simulink model "PHRI_MODEL_PROJECT"  (R2020b)
settings: Solver=VariableStepAuto  StartTime=0.0  StopTime=20  RelTol=1e-3
values from neighbouring files (symbols this model uses):
  A = [1 Ts;0 1]    [parameters.m]
  Be = 1    [parameters.m]
  beta = 2*pi*Fc*Ts / (1+2*pi*Fc*Ts)    (= 0.111635211705)    [parameters.m]
  Bh = 0.02    [parameters.m]
  Bh_hat = 0.05    [parameters.m]
  C = [1 0]    [parameters.m]
  delayCommM2S = 400    [parameters.m]
  delayCommS2M = 400    [parameters.m]
  Fc = 20    [parameters.m]
  Fc_h = 1    [parameters.m]
  Jh = 0.00002    (= 2e-05)    [parameters.m]
  k_m = 19.34    [parameters.m]
  k_s = 19.34    [parameters.m]
  Kc2v_m = 2    [parameters.m]
  Kc2v_s = 2    [parameters.m]
  Kd_h = 1.125    [parameters.m]
  Kd_m = 1.5    [parameters.m]
  Kd_s = 1.5    [parameters.m]
  Ke = 10    [parameters.m]
  Kh_hat = 1    [parameters.m]
  Kh_max = 50    [parameters.m]
  Kp_h = 1    [parameters.m]
  Kp_m = 1    [parameters.m]
  Kp_s = 1    [parameters.m]
  Kt2c_m = 1.182    [parameters.m]
  Kt2c_s = 1.182    [parameters.m]
  lArm_m = 0.1    [parameters.m]
  lArm_s = 0.1    [parameters.m]
  maxCurrent_m = 4.5    [parameters.m]
  maxCurrent_s = 4.5    [parameters.m]
  PosRef = 1    [parameters.m]
  qe = 2    [parameters.m]
  stopTime = str2double(stopTime)    [parameters.m]
  tau_m = 1.217    [parameters.m]
  tau_s = 1.217    [parameters.m]
  Ts = 0.001    [parameters.m]
  Variance = 0.0000001    (= 1e-07)    [parameters.m]
undefined symbols (not defined in the file or in its folder): DiscIntNeverNeededParam, Discrete, Time
libraries: simulink_extras x37, dspsigops x37, ctrlSharedLib x16, cstblocks x1
(part 3 of 3)

== matlab function PHRI_MODEL_PROJECT/MASTER SIDE/Velocity Approx + LPF 3/Euler Approximation  ==
  data: beta input; Ts input; filtered output; pos input; posPrev input; filteredPrev input
function filtered = EulApprox(beta, Ts, pos, posPrev, filteredPrev)

eul= (pos - posPrev)/Ts;
filtered = beta*eul + (1-beta)*filteredPrev;

== matlab function PHRI_MODEL_PROJECT/MASTER SIDE1/Euler Approximation Vel MH2/Euler Approximation  ==
  data: beta input; Ts input; filtered output; pos input; posPrev input; filteredPrev input
function filtered = EulApprox(beta, Ts, pos, posPrev, filteredPrev)

eul= (pos - posPrev)/Ts;
filtered = beta*eul + (1-beta)*filteredPrev;

== matlab function PHRI_MODEL_PROJECT/Euler Approximation Vel M1/Euler Approximation  ==
  data: beta input; Ts input; filtered output; pos input; posPrev input; filteredPrev input
function filtered = EulApprox(beta, Ts, pos, posPrev, filteredPrev)

eul= (pos - posPrev)/Ts;
filtered = beta*eul + (1-beta)*filteredPrev;

== matlab function PHRI_MODEL_PROJECT/SLAVE_SIDE /Velocity Approx + LPF 3/Euler Approximation  ==
  data: beta input; Ts input; filtered output; pos input; posPrev input; filteredPrev input
function filtered = EulApprox(beta, Ts, pos, posPrev, filteredPrev)

eul= (pos - posPrev)/Ts;
filtered = beta*eul + (1-beta)*filteredPrev;
